simulink model "AB2Auf2simlnk"  (R2024b)
settings: Solver=ode4  StartTime=0.0  StopTime=12  FixedStep=0.01  RelTol=1e-3
values from neighbouring files (symbols this model uses):
  A = [0        -(k1+k2)/m1     0            k2/m1;      1        0               0            0;      0        k2/m2           0            -(k2+k3)/m2;      0        0               1            0]    [AB1Auf2.m]    (also in AB1Auf4.m = [ -0.05    -0.003     -0.98      0.2;       -1       -0.75  ; AB2Auf2.m = [-2 1 0; -10 0 -15; 0 1 0]; AB3Auf1.m = [Y_beta/u0 -(1-Y_r/u0); N_beta N_r])
  B = [0 0; 1.7 -0.2; 0.3 -0.6; 0 0]    [AB1Auf4.m]    (also in AB2Auf2.m = [0; -5; 0]; AB3Auf1.m = [Y_del_rud;N_del_rud])
  C = eye(size(A))    [AB1Auf4.m]    (also in AB2Auf2.m = eye(3,3); AB3Auf1.m)
  D = zeros(size(B))    [AB1Auf4.m]    (also in AB2Auf2.m = zeros(3,1); AB3Auf1.m; AB5Auf1.m = a1 ./ (2 * Omega_0); AB6.m = -real(L(1)) / omega_0)
settings Model: Creator=the_main_notebook  LastModifiedBy=the_main_notebook

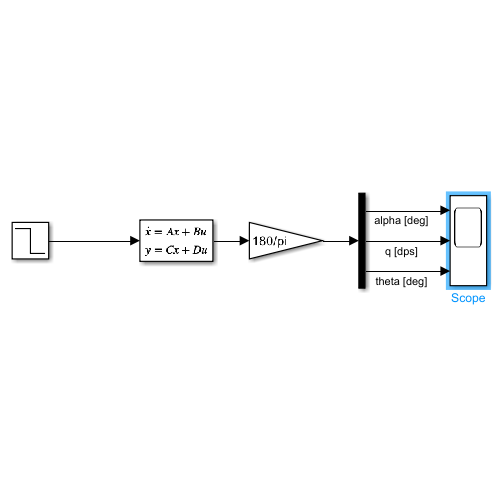
[thumbnail: Simulink's stored preview of the top-level diagram]
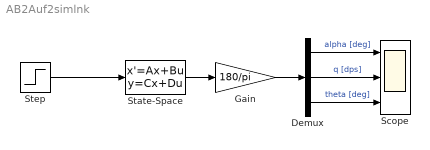
== system AB2Auf2simlnk ==
  Demux : Demux  Outputs=3
  Gain : Gain  Gain=180/pi
  Scope : Scope  NumInputPorts=3
  State-Space : StateSpace  A=A  B=B  C=C  D=D  InitialCondition=0
  Step : Step  Time=2  After=deg2rad(-3)  SampleTime=0
  wires:
  State-Space/1 -> Gain/1
  Step/1 -> State-Space/1
  Gain/1 -> Demux/1
  Demux/1 -> Scope/1  "alpha [deg]"
  Demux/2 -> Scope/2  "q [dps]"
  Demux/3 -> Scope/3  "theta [deg]"
